simulink model "c2838xd_ipc_cm"  (R2021b)
settings: Solver=FixedStepDiscrete  StartTime=0.0  StopTime=Inf  RelTol=1e-3  EnableMultiTasking=on
libraries: c2838x_M4_lib x8, demo_controls x1
settings Model: SimulationMode=external  Creator=The MathWorks, Inc.  LastModifiedBy=The MathWorks, Inc.
settings SolverCC: AlgebraicLoopSolver=TrustRegion  AutoInsertRateTranBlk=on  MinimalZcImpactIntegration=on
settings DataIOCC: ReturnWorkspaceOutputs=off
settings OptimizationCC: DefaultUnderspecifiedDataType=single  EnhancedBackFolding=on  StrengthReduction=on  PassReuseOutputArgsAs=Individual arguments  ZeroExternalMemoryAtStartup=off  MaxStackSize=2560  OptimizeBlockOrder=speed  DifferentSizesBufferReuse=on  DenormalBehavior=FlushToZero  EfficientTunableParamExpr=on
settings DebuggingCC: ParameterTunabilityLossMsg=error  SFMachineParentedDataDiag=warning  ArithmeticOperatorsInVariantConditions=warning
settings HardwareCC: ProdBitPerPointer=32  ProdBitPerSizeT=32  ProdBitPerPtrDiffT=32  ProdLargestAtomicInteger=Long  ProdLargestAtomicFloat=Double  ProdWordSize=32  ProdLongLongMode=on  ProdHWDeviceType=ARM Compatible->ARM Cortex
settings SFSimCC: SimUseLocalCustomCode=off  MATLABDynamicMemAlloc=off  CustomCodeUndefinedFunction=UseInterfaceOnly
settings RTWCC: Description=Embedded Coder  SystemTargetFile=ert.tlc  HardwareBoard=TI F2838x (ARM Cortex-M4)  TemplateMakefile=ert_default_tmf  GenerateReport=on  RTWUseLocalCustomCode=off  Toolchain=Texas Instruments Code Composer Studio (ARM)  BuildConfiguration=Debug  IncludeHyperlinkInReport=on  LaunchReport=on  GenerateTraceInfo=on  GenerateTraceReport=on  GenerateTraceReportSl=on  GenerateTraceReportSf=on  GenerateTraceReportEml=on
settings CodeAppCC: ForceParamTrailComments=on  IgnoreCustomStorageClasses=off  OperatorAnnotations=on  SimulinkDataObjDesc=on  SFDataObjDesc=on  InsertBlockDesc=on
settings ERTTargetCC: ExtModeStaticAllocSize=10000

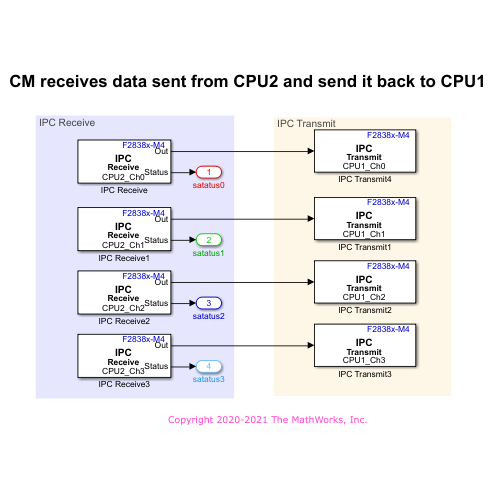
[thumbnail: Simulink's stored preview of the top-level diagram]
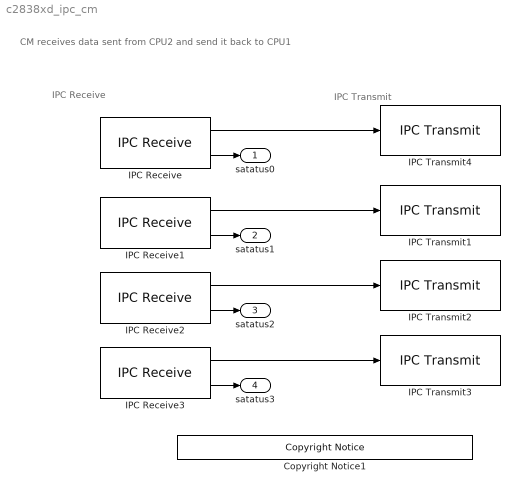
== system c2838xd_ipc_cm ==
  note: IPC Receive
  note: IPC Transmit
  note: CM receives data sent from CPU2 and send it back to CPU1
  Copyright Notice1 : demo_controls/Copyright Notice  year=2020  prod=tic2000
      settings: SourceProductBaseCode=ME
  IPC Receive : c2838x_M4_lib/IPC Receive  SelectSource=CPU2  SelectChannel=0  DataType=uint16  DataLength=1  EnableBlocking=off  SampleTime=0.25
      settings: SourceProductBaseCode=TIC2000
  IPC Receive1 : c2838x_M4_lib/IPC Receive  SelectSource=CPU2  SelectChannel=1  DataType=uint16  DataLength=1  EnableBlocking=off  SampleTime=0.5
      settings: SourceProductBaseCode=TIC2000
  IPC Receive2 : c2838x_M4_lib/IPC Receive  SelectSource=CPU2  SelectChannel=2  DataType=uint16  DataLength=1  EnableBlocking=off  SampleTime=1
      settings: SourceProductBaseCode=TIC2000
  IPC Receive3 : c2838x_M4_lib/IPC Receive  SelectSource=CPU2  SelectChannel=3  DataType=uint16  DataLength=1  EnableBlocking=off  SampleTime=2
      settings: SourceProductBaseCode=TIC2000
  IPC Transmit1 : c2838x_M4_lib/IPC Transmit  SelectDestination=CPU1  SelectChannel=1  EnableBlocking=off
      settings: SourceProductBaseCode=TIC2000
  IPC Transmit2 : c2838x_M4_lib/IPC Transmit  SelectDestination=CPU1  SelectChannel=2  EnableBlocking=off
      settings: SourceProductBaseCode=TIC2000
  IPC Transmit3 : c2838x_M4_lib/IPC Transmit  SelectDestination=CPU1  SelectChannel=3  EnableBlocking=off
      settings: SourceProductBaseCode=TIC2000
  IPC Transmit4 : c2838x_M4_lib/IPC Transmit  SelectDestination=CPU1  SelectChannel=0  EnableBlocking=off
      settings: SourceProductBaseCode=TIC2000
  satatus0 : Outport
  satatus1 : Outport  Port=2
  satatus2 : Outport  Port=3
  satatus3 : Outport  Port=4
  wires:
  IPC Receive/1 -> IPC Transmit4/1
  IPC Receive1/1 -> IPC Transmit1/1
  IPC Receive2/1 -> IPC Transmit2/1
  IPC Receive3/1 -> IPC Transmit3/1
  IPC Receive/2 -> satatus0/1
  IPC Receive1/2 -> satatus1/1
  IPC Receive2/2 -> satatus2/1
  IPC Receive3/2 -> satatus3/1
